simulink library "epoch_time_lib"  (R2016a)
settings: Solver=ode45  StartTime=0.0  StopTime=10.0  RelTol=1e-3
undefined symbols (not defined in the file): ARMdT, DiscIntNeverNeededParam, slowARMdT
libraries: simulink x1
settings Model: Creator=ch24070  LastModifiedBy=CH24070
settings DataIOCC: LimitDataPoints=on
settings DebuggingCC: AllowSymbolicDim=off

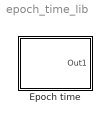
== system epoch_time_lib ==
  Epoch time : Subsystem  mask{syncRate=slowARMdT*100, clkRate=ARMdT}
      mask prompts: syncRate "Rate to sync to OS clock"; clkRate "Rate to update clock output"

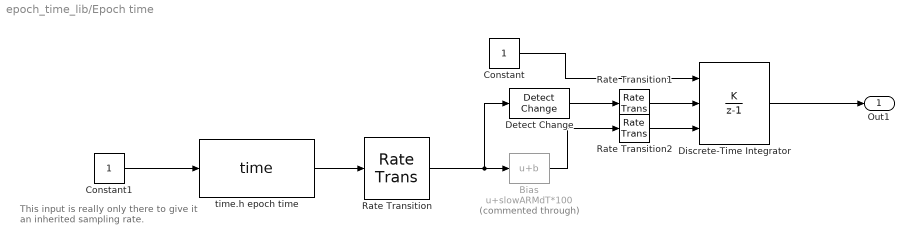
== system epoch_time_lib/Epoch time ==
  note: This input is really only there to
      |  give it an inherited sampling rate.
  Bias : Bias  Commented=through  Bias=slowARMdT*100
  Constant : Constant
  Constant1 : Constant  SampleTime=syncRate
  Detect Change : simulink/Logic and Bit Operations/Detect Change  vinit=0  OutDataTypeStr=boolean
  Discrete-Time Integrator : DiscreteIntegrator  IntegratorMethod=Accumulation: Forward Euler  gainval=clkRate  ExternalReset=rising  InitialConditionSource=external  InitialConditionSetting=State (most efficient)  SampleTime=clkRate  OutDataTypeStr=double  ICPrevOutput=DiscIntNeverNeededParam  ICPrevScaledInput=DiscIntNeverNeededParam
  Rate Transition : RateTransition  OutPortSampleTime=syncRate
  Rate Transition1 : RateTransition  Deterministic=off  OutPortSampleTime=clkRate
  Rate Transition2 : RateTransition  Deterministic=off  OutPortSampleTime=clkRate
  time.h epoch time : S-Function  InitFcn=try, set_param(gcb,'FunctionName','time'), end  FunctionName=time  SFunctionModules=time_wrapper  SFunctionDeploymentMode=off  EnableBusSupport=off  mask(S-Function Builder){}
      mask help: Simulink:masks:SFunctionBuilder_MD
      mask init:
      | val = [[.9  0.75 0.75 1 1 .9 .9 1]',[1 1 0.75 0.75 .9 .9 1 .9]'];try , sys = get_param(gcb,'SfunBuilderFcnName');if isempty(sys), sys = get_param(gcb,'FunctionName'); end,catch, sys = get_param(gcb,'FunctionName'); end
      settings: PreSaveFcn=try, set_param(gcb,'FunctionName','time'), end  OpenFcn=sfunctionwizard(gcbh)
      mask Display: plot(val(:,1),val(:,2)),disp(sys), port_label('input',1,'dummy'), port_label('output',1,'y0')
  Out1 : Outport
  wires:
  Constant1/1 -> time.h epoch time/1
  Rate Transition2/1 -> Discrete-Time Integrator/3
  Rate Transition1/1 -> Discrete-Time Integrator/2
  time.h epoch time/1 -> Rate Transition/1
  Rate Transition/1 -> Bias/1, Detect Change/1
  Constant/1 -> Discrete-Time Integrator/1
  Discrete-Time Integrator/1 -> Out1/1
  Detect Change/1 -> Rate Transition1/1
  Bias/1 -> Rate Transition2/1
